simulink library "pwrsysBasic"  (R2016a)
settings: Solver=VariableStepAuto  SolverMode=SingleTasking  StartTime=0.0  StopTime=10.0  RelTol=1e-3
values from neighbouring files (symbols this model uses):
  Ts = Ts_c    (= 1e-07)    [PlantStateEquations_abc_Script.m]
undefined symbols (not defined in the file or in its folder): DiscIntNeverNeededParam, fn, Iap, Uanp
undefined symbols (not defined in the file): Sn, tctrl
libraries: pwrsysBasic x15, powerlib_meascontrol x12, pwrsysTransf x8, simulink x2
(part 1 of 2)
settings Model: Creator=daniemot  LastModifiedBy=daniemot
settings DebuggingCC: SFUnexpectedBacktrackingDiag=error  SFNoUnconditionalDefaultTransitionDiag=error
settings GRTTargetCC: TargetLangStandard=C99 (ISO)  GeneratePreprocessorConditionals=Use local settings
settings ConfigComp: CovMetricSettings=dwe  CovHtmlReporting=off  CovSaveCumulativeToWorkspaceVar=off  CovSaveSingleToWorkspaceVar=off  CovExternalEMLEnable=on

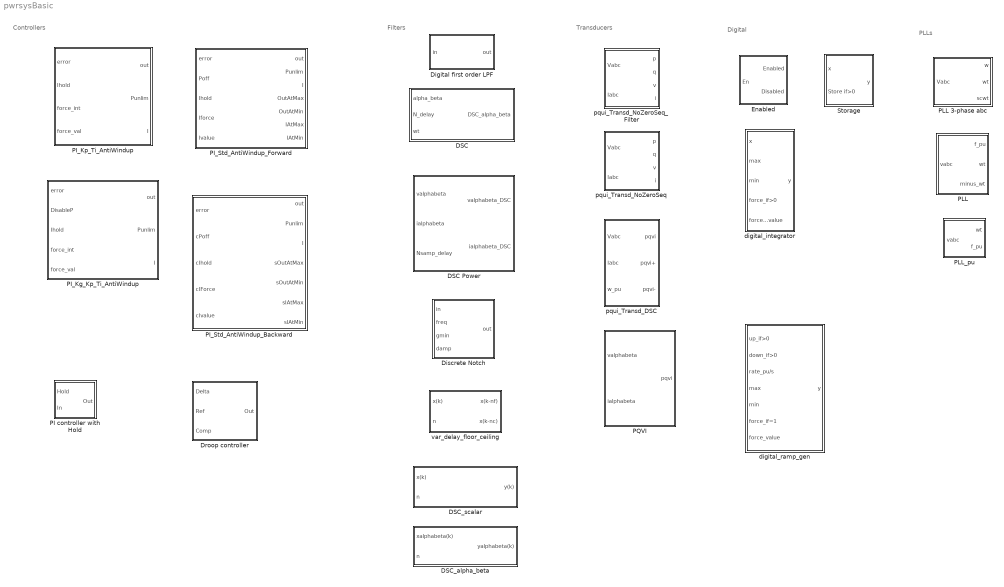
== system pwrsysBasic ==
  note: PLLs
  note: Controllers
  note: Filters
  note: Transducers
  note: Digital
  DSC : Subsystem
  "DSC Power " : Subsystem
  DSC_alpha_beta : Subsystem  mask(Delayed signal cancellation of a scalar){nmax=200}
      mask prompts: nmax "Circular buffer size"
      mask help: Performs an adaptive delayed signal cancellation of the input x. The input n should be equal to (floating point) number of samples corresponding to half the period of the frequency f one intends to filter.
      mask Help:
      | Performs two delayed signal cancellation of the input x:
      | 	yf(k) = 0.5 (x(k) + x(k-nf(k))
      | 	yc(k) = 0.5 (x(k) + x(k-nc(k))
      | where, f stands for floor and c for ceiling.
      | 
      | The two values yf and yc are then weigthed according to how far the real value n is from nc or nf.
      | 
      | Inputs:
      | 	x: input signal
      | 	n: floating point representing the number of samples equal to half the period of the frequecy one intends to suppress
      | 
      | Output:
      | 	y: output with the delayed signal cancelled value of the input
      | 
      | Parameter:
      | 	Circular buffer size: set to the number of samples that corresponds to half the period of the lowest frequency one intends to filter.
      | 
      | States:
      | 	Uses an S-function with a circular buffer that supplies the delayed (ceiling and floor of n) values of the input.
      mask Display: fprintf('DSC');
  DSC_scalar : Subsystem  mask(Delayed signal cancellation of a scalar){nmax=200}
      mask prompts: nmax "Circular buffer size"
      mask help: Performs an adaptive delayed signal cancellation of the input x. The input n should be equal to (floating point) number of samples corresponding to half the period of the frequency f one intends to filter.
      mask Help:
      | Performs two delayed signal cancellation of the input x:
      | 	yf(k) = 0.5 (x(k) + x(k-nf(k))
      | 	yc(k) = 0.5 (x(k) + x(k-nc(k))
      | where, f stands for floor and c for ceiling.
      | 
      | The two values yf and yc are then weigthed according to how far the real value n is from nc or nf.
      | 
      | Inputs:
      | 	x: input signal
      | 	n: floating point representing the number of samples equal to half the period of the frequecy one intends to suppress
      | 
      | Output:
      | 	y: output with the delayed signal cancelled value of the input
      | 
      | Parameter:
      | 	Circular buffer size: set to the number of samples that corresponds to half the period of the lowest frequency one intends to filter.
      | 
      | States:
      | 	Uses an S-function with a circular buffer that supplies the delayed (ceiling and floor of n) values of the input.
      mask Display: fprintf('y(k)=0.5(x(k) + x(k-n))');
  Digital first order LPF : Subsystem  mask(Digital first-order low-pass filter){Ts=tctrl, fcutout=fn/2^0.5}
      mask prompts: Ts "Sample times [s]"; fcutout "Cutout frequency [Hz]"
      mask help:
      | Continuous time transfer function:  1/(1 + s T)
      | 	where T [s] = 1 / (2 pi fcutout [Hz]).
      |
      | Actual digital transfer function:   alpha / (1 + ( alpha -1) z^{-1} )
      | 	with eq. of diffs.: y = alpha x + (1 - alpha) y z^{-1}
      | 	where alpha = Ts / ( 1/(2 pi fcutout) + Ts)
      mask Display: fprintf('1/(1+sT)');
  Discrete Notch : Subsystem  TreatAsAtomicUnit=on  mask(Discrete Notch with time-varying parameters){Ts=0.001}
      mask prompts: Ts "Sample time Ts (s)"
      mask help:
      | The block implements the Tustin discretization of a continuous-time notch filter with time-varying coefficients:
      | (s^2+2*gmin*damp*freq*s+freq^2)/(s^2+2*damp*freq*s+freq^2)
      |
      | Parameters:
      | - freq is the notch frequency (rad/s)
      | - gmin is the minimum gain
      | - damp is the damping ratio
      mask Display: fprintf('notch');
  Droop controller : Subsystem  mask(Droop controller){Refmax=1, Refmin=-1, Ts=-1, Kp=1, Kd=0, Tr=0.1, flp=100, DB=0}
      mask prompts: Refmax "Max reference"; Refmin "Min reference"; Ts "Sample time"; Kp "Permanent gain"; Kd "Transient gain"; Tr "Reset time [s]"; flp "Low-pass filter cut-off frequency [Hz]"; DB "Dead-band"
      mask help:
      | This block implements a droop controller, i.e. it provides compensation of the input Ref based on the input Delta and Comp.
      |
      | The input Delta is used as input of a PD controller which provides permanent (proportional) and transient (derivative) droop of the input Ref.
      |
      | The input Comp divides the output value of the droop controller and may be used for other types of compensation.
      mask DialogControl DescTextVar Prompt: This block implements a simplified model for power control with droop influence. It can be used either for active power with frequency droop influence or reactive power with voltage droop influence.
  Enabled : Subsystem  SystemSampleTime=Ts  mask(Enabled block){}
      mask help:
      | if En > 0
      |     Enabled = 1;
      |     Disabled = 0;
      | else
      |     Enabled = 0;
      |     Disabled = 1;
      | end
      mask Display: fprintf('Enable');
  PI controller with Hold : Subsystem  mask(PI controller with anti-windup){Kp=1, Ki=0, Max=1, Min=-1, x0=0, Ts=1e-4}
      mask prompts: Kp "Proportional gain"; Ki "Integral gain"; Max "Maximum output"; Min "Minimum output"; x0 "Initial condition"; Ts "Sampling time"
      mask help:
      | This block implements a PI controller with anti-windup
      |
      | The input hold freezes the integrator and allows implementing anti-windup in control loops with feed-forward or dynamic limits
  PI_Kg_Kp_Ti_AntiWindup : Subsystem  TreatAsAtomicUnit=on  SystemSampleTime=Ts  mask(PI regulator with anti-windup){Ts=0.001, Kg=1, Kp=1, Ti=1, PI_max=1, PI_min=-1}
      mask prompts: Ts "Sampling time [s]"; Kg "Loop gain: Kg [pu]"; Kp "Proportional gain: Kp [pu]"; Ti "Integral time: Ti [s]"; PI_max "Maximum output [pu]"; PI_min "Minimum output [pu]"
      mask help:
      | Discrete PI regulator with forward Euler approximation for the integrator.
      |
      | Transfer function:
      | 	Kg (Kp + 1/sTi)
      |
      | The anti-windup freezes the integrator if the unlimited output of the PI goes beyond the limits.
      |
      | It is possible to disable the proportional (Kp) contribution.
      settings: MinAlgLoopOccurrences=on
      mask Display: fprintf('Kg(Kp+1/(sTi))');
  PI_Kp_Ti_AntiWindup : Subsystem  TreatAsAtomicUnit=on  SystemSampleTime=Ts  mask(PI regulator with anti-windup){Ts=0.001, Kp=10, Ti=1, PI_max=1, PI_min=-1}
      mask prompts: Ts "Sampling time [s]"; Kp "Proportional gain: Kp [pu]"; Ti "Integral time: Ti [s]"; PI_max "Maximum output [pu]"; PI_min "Minimum output [pu]"
      mask help:
      | Discrete PI regulator with forward Euler approximation for the integrator.
      |
      | Transfer function:
      | 	Kp (1 + sTi) / (sTi)
      |
      | The anti-windup freezes the integrator if the unlimited output of the PI goes beyond the limits.
      settings: MinAlgLoopOccurrences=on
      mask Display: fprintf('Kp(1+1/(sTi))');
  PI_Std_AntiWindup_Backward : Subsystem  mask(PI regulator with anti-windup){Ts=1, Kg=1, Kp=1, Ti=1, outMax=1, outMin=1}
      mask prompts: Ts "Sampling time [s]"; Kg "Loop gain Kg [pu]"; Kp "Proportional gain Kp [pu]"; Ti "Integral time Ti [s]"; outMax "Maximum output [pu]"; outMin "Minimum output [pu]"
      mask help:
      | Discrete PI regulator in standard form with loop gain and backward Euler approximation.
      |
      | Transfer function:
      | 	Kg (Kp + 1/sTi)
      |
      | The anti-windup freezes the integrator if the unlimited output of the PI goes beyond the limits.
      |
      | It is possible to:
      | - Disable the proportional (Kp) contribution. (Poff > 0)
      | - Freeze the integrator (Ihold >0)
      | - Force the integrator to Ivalue (Iforce >0)
      mask Display: fprintf('Kg(Kp+1/(sTi))');
  PI_Std_AntiWindup_Forward : Subsystem  SystemSampleTime=Ts  mask(PI regulator with anti-windup){Ts=0.001, Kg=1, Kp=1, Ti=1, outMax=1, outMin=-1}
      mask prompts: Ts "Sampling time [s]"; Kg "Loop gain: Kg [pu]"; Kp "Proportional gain: Kp [pu]"; Ti "Integral time: Ti [s]"; outMax "Maximum output [pu]"; outMin "Minimum output [pu]"
      mask help:
      | Discrete PI regulator in standard form with loop gain and forward Euler method  for the integrator.
      |
      | Transfer function:
      | 	Kg (Kp + 1/sTi)
      |
      | The anti-windup freezes the integrator if the unlimited output of the PI goes beyond the limits.
      |
      | It is possible to:
      | - Disable the proportional (Kp) contribution. (Poff > 0)
      | - Freeze the integrator (Ihold >0)
      | - Force the integrator to Ivalue (Iforce >0)
      settings: MinAlgLoopOccurrences=on
      mask Display: fprintf('Kg(Kp+1/(sTi))');
  PLL : Subsystem  mask(Matlabs PLL with POS and NEG omega t output){fn=0, Ts=0.00005, Kp_pll=90, Ki_pll=1600, Kd_pll=0, PLL_ini=0}
      mask prompts: fn "Rated frequency [Hz]"; Ts "Sampling time [s]"; Kp_pll "Proportional gain: Kp_pll"; Ki_pll "Integral gain: Ki_pll"; Kd_pll "Derivative gain: Kd_pll"; PLL_ini "PLL initial angle: PLL_ini [degrees]"
  PLL 3-phase abc : Subsystem  mask(3-Phase PLL in the abc frame){fnom=50, fdev=20, zeta=0.707, Kp=100, Ki=50, Kd=1e4, Tr=100, Ts=1e-4, wt0=0}
      mask prompts: fnom "Rated frequency [Hz]"; fdev "Maximum frequency deviation [Hz]"; zeta "Damping ratio"; Kp "Proportional gain"; Ki "Integral gain"; Kd "Derivative gain"; Tr "Reset time [s]"; Ts "Sampling time [s]"; wt0 "Initial angle [rad/s]"
      mask help: This block implements a 3-phase PLL in the abc reference frame.
      mask init:
      | wn = fnom/(4*zeta);
      mask DialogControl freqFilter Prompt: Frequency filter
      mask DialogControl ctrl Prompt: Controller
  PLL_pu : Subsystem  mask(Matlabs PLL with POS and NEG omega t output){fn=50, Ts=100e-6, Kp_pll=90, Ki_pll=1600, Kd_pll=0, PLL_ini=0}
      mask prompts: fn "Rated frequency [Hz]"; Ts "Sampling time [s]"; Kp_pll "Proportional gain: Kp_pll"; Ki_pll "Integral gain: Ki_pll"; Kd_pll "Derivative gain: Kd_pll"; PLL_ini "PLL initial angle: PLL_ini [degrees]"
  PQVI : Subsystem  mask(u i p q transducer - No zero sequence){Sn=Sn, Uanp=Uanp, Iap=Iap}
      mask prompts: Sn "Rated three-phase apparent power [VA]"; Uanp "Rated peak phase-to-groud voltage [V]"; Iap "Rated peak line current [A]"
      mask help:
      | Loosely based on Akagi 1984, but with Clarke Transformation for both the current and voltage
      | 	v  = (valpha^2 + vbeta^2)^0.5 / V_phase_peak
      | 	i   = (ialpha^2 + ibeta^2)^0.5 / I_line_peak
      | 	p  = 3/2 * (valpha ialpha +vbeta ibeta) / Sn
      | 	q  = 3/2 * (-valpha ibeta +vbeta ialpha) / Sn
  Storage : Subsystem  SystemSampleTime=Ts  mask(Storage block){}
      mask help:
      | if Store ==1
      |     Output = Input;
      | else
      |     Output = old ouptut;
      | end
      mask Display: fprintf('Store');
  digital_integrator : Subsystem  SystemSampleTime=Ts  mask(Digital integrator){Ts=Ts}
      mask prompts: Ts "Sample times [s]"
      mask help:
      | Forward Euler method: as in matlab help
      | 	y(n) = y(n-1) + Ts(n-1)*x(n-1)
      | uset it to avoid algebraic loops
      |
      | All inputs are stored in states, so there is no direct feedthrough. GAMBIARRA for avoiding algebraic loops, see https://www.mathworks.com/help/simulink/ug/integration-considerations-for-matlab-function-blocks.html
      |
      | Inputs
      |    x: input to the integrator
      |    max: max value for integrator
      |    min: min value for integrator
      |    force: if>=1 sets integrator to forceval
      |    forceval: see line above (max and min are respected
      |    Ts: sampling time
      | Output
      |    y: output of the integrator
      mask Display: fprintf('1/s');
  digital_ramp_gen : Subsystem  SystemSampleTime=Ts  mask(Digital ramp generator){Ts=tctrl}
      mask prompts: Ts "Sample times [s]"
      mask help: Allways starts at zero. Can be forced to a value, and will stay there, but in the first two cycles will stay at zero.
      mask Display: fprintf('Ramp');
  pqui_Transd_DSC : Subsystem  mask(DSC u i p q transducer - No zero sequence){Ts=0.000005, fn=50, Sn=Sn, Uanp=Uanp, Iap=Iap}
      mask prompts: Ts "Sampling time [s]"; fn "Rated frequency [Hz]"; Sn "Rated three-phase apparent power [VA]"; Uanp "Rated peak phase-to-groud voltage [V]"; Iap "Rated peak line current [A]"
      mask help:
      | Loosely based on Akagi 1984, but with Clarke Transformation for both the current and voltage
      | 	v  = (valpha^2 + vbeta^2)^0.5 / V_phase_peak
      | 	i   = (ialpha^2 + ibeta^2)^0.5 / I_line_peak
      | 	p  = 3/2 * (valpha ialpha +vbeta ibeta) / Sn
      | 	q  = 3/2 * (-valpha ibeta +vbeta ialpha) / Sn
  pqui_Transd_NoZeroSeq : Subsystem  mask(u i p q transducer - No zero sequence){Sn=Sn, Uanp=Uanp, Iap=Iap}
      mask prompts: Sn "Rated three-phase apparent power [VA]"; Uanp "Rated peak phase-to-groud voltage [V]"; Iap "Rated peak line current [A]"
      mask help:
      | Loosely based on Akagi 1984, but with Clarke Transformation for both the current and voltage
      | 	v  = (valpha^2 + vbeta^2)^0.5 / V_phase_peak
      | 	i   = (ialpha^2 + ibeta^2)^0.5 / I_line_peak
      | 	p  = 3/2 * (valpha ialpha +vbeta ibeta) / Sn
      | 	q  = 3/2 * (-valpha ibeta +vbeta ialpha) / Sn
  pqui_Transd_NoZeroSeq_Filter : Subsystem  mask(u i p q transducer - No zero sequence){Ts=0.001, Sn=1000, fn=50, Uanp=1000, Iap=1000, fcutoutvi=1000, fcutoutpq=1000, zeta=0.7}
      mask prompts: Ts "Sampling time [s]"; Sn "Rated three-phase apparent power [VA]"; fn "Rated frequency [Hz]"; Uanp "Rated peak phase-to-groud voltage [V]"; Iap "Rated peak line current [A]"; fcutoutvi "Cutout freq. low-pass for v&i meas. [Hz]"; fcutoutpq "Cutout freq. low-pass for p&q meas. [Hz]"; zeta "Zeta for all second order filters"
      mask help:
      | Loosely based on Akagi 1984, but with Clarke Transformation for both the current and voltage
      | 	v  = (valpha^2 + vbeta^2)^0.5 / V_phase_peak
      | 	i   = (ialpha^2 + ibeta^2)^0.5 / I_line_peak
      | 	p  = 3/2 * (valpha ialpha +vbeta ibeta) / Sn
      | 	q  = 3/2 * (-valpha ibeta +vbeta ialpha) / Sn
      |
      | Second order low-pass filter for all measurements
      |
      | Notch filter at the rated frequency
  var_delay_floor_ceiling : Subsystem  mask(Circular buffer with two variable delays (ceiling and floor)){nmax=40}
      mask prompts: nmax "Circular buffer size"
      mask help: Provides the values of the input delayed by floor(n) and ceil(n) samples.
      mask Help:
      | Provides the values of the input delayed by floor(n) and ceil(n) samples.
      | 
      | S-Function source code:
      | 	variable_delay_floor_ceil.c
      | 	variable_delay_floor_ceil_wrapper.c
      | 	variable_delay_floor_ceil.tlc
      | 
      | mexw64:
      | 	variable_delay_floor_ceil.mexw64
      | 
      | The mex file can be regenerated by running this at the command line:
      | 	mex variable_delay_floor_ceil.c variable_delay_floor_ceil_wrapper.c
      | This assumes that the addons for compiling are installed.

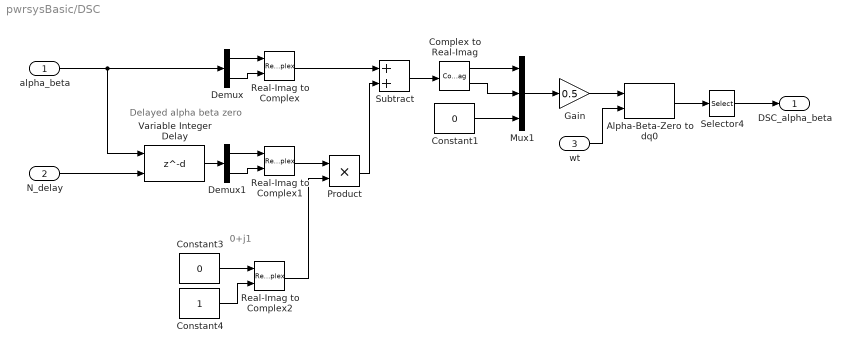
== system pwrsysBasic/DSC ==
  note: 0+j1
  note: Delayed alpha beta zero
  alpha_beta : Inport
  N_delay : Inport  Port=2
  wt : Inport  Port=3
  Alpha-Beta-Zero to dq0 : powerlib_meascontrol/Transformations/Alpha-Beta-Zero to dq0  Alignment=90 degrees behind phase A axis
  Complex to Real-Imag : ComplexToRealImag
  Constant1 : Constant  Value=0
  Constant3 : Constant  Value=0
  Constant4 : Constant
  Demux : Demux  Outputs=2
  Demux1 : Demux  Outputs=2
  Gain : Gain  Gain=0.5
  Mux1 : Mux  Inputs=[1 1 1]
  Product : Product
  Real-Imag to Complex : RealImagToComplex
  Real-Imag to Complex1 : RealImagToComplex
  Real-Imag to Complex2 : RealImagToComplex
  Selector4 : Selector  InputPortWidth=3  IndexOptions=Index vector (dialog)  Indices=[1 2]  OutputSizes=1
  Subtract : Sum
  Variable Integer Delay : Delay  DelayLengthSource=Input port  DelayLength=200  DelayLengthUpperLimit=500  SampleTime=Ts
      settings: InputPortMap=u0,p1
  DSC_alpha_beta : Outport
  wires:
  Product/1 -> Subtract/2
  Demux/1 -> Real-Imag to Complex/1
  Real-Imag to Complex1/1 -> Product/1
  Demux1/1 -> Real-Imag to Complex1/1
  wt/1 -> Alpha-Beta-Zero to dq0/2
  Complex to Real-Imag/1 -> Mux1/1
  Variable Integer Delay/1 -> Demux1/1
  Demux1/2 -> Real-Imag to Complex1/2
  N_delay/1 -> Variable Integer Delay/2
  Gain/1 -> Alpha-Beta-Zero to dq0/1
  Constant3/1 -> Real-Imag to Complex2/1
  Real-Imag to Complex/1 -> Subtract/1
  alpha_beta/1 -> Variable Integer Delay/1, Demux/1
  Real-Imag to Complex2/1 -> Product/2
  Subtract/1 -> Complex to Real-Imag/1
  Constant1/1 -> Mux1/3
  Demux/2 -> Real-Imag to Complex/2
  Constant4/1 -> Real-Imag to Complex2/2
  Complex to Real-Imag/2 -> Mux1/2
  Mux1/1 -> Gain/1
  Alpha-Beta-Zero to dq0/1 -> Selector4/1
  Selector4/1 -> DSC_alpha_beta/1

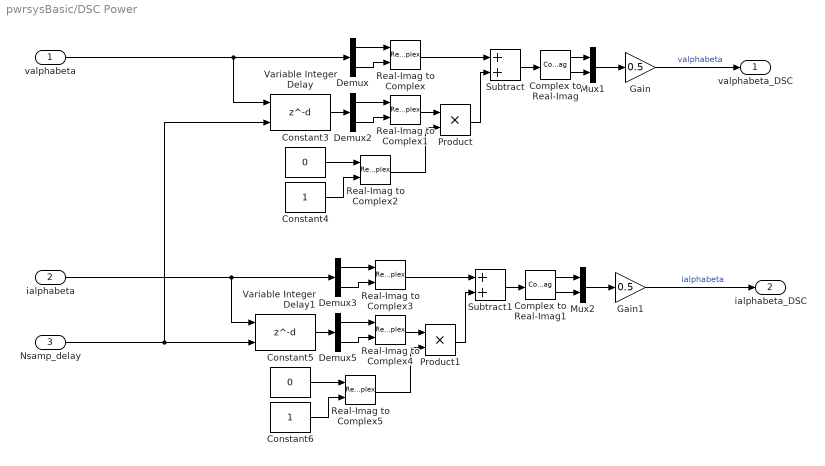
== system pwrsysBasic/DSC Power  ==
  valphabeta : Inport
  ialphabeta : Inport  Port=2
  Nsamp_delay : Inport  Port=3
  Complex to Real-Imag : ComplexToRealImag
  Complex to Real-Imag1 : ComplexToRealImag
  Constant3 : Constant  Value=0
  Constant4 : Constant
  Constant5 : Constant  Value=0
  Constant6 : Constant
  Demux{,2..3,5} (4 alike) : Demux  Outputs=2
  Gain : Gain  Gain=0.5
  Gain1 : Gain  Gain=0.5
  Mux1 : Mux  Inputs=[1 1]
  Mux2 : Mux  Inputs=[1 1]
  Product : Product
  Product1 : Product
  Real-Imag to Complex{,1..5} (6 alike) : RealImagToComplex
  Subtract : Sum
  Subtract1 : Sum
  Variable Integer Delay : Delay  DelayLengthSource=Input port  DelayLength=200  DelayLengthUpperLimit=500  SampleTime=Ts
      settings: InputPortMap=u0,p1
  Variable Integer Delay1 : Delay  DelayLengthSource=Input port  DelayLength=200  DelayLengthUpperLimit=500  SampleTime=Ts
      settings: InputPortMap=u0,p1
  valphabeta_DSC : Outport
  ialphabeta_DSC : Outport  Port=2
  wires:
  Demux2/2 -> Real-Imag to Complex1/2
  Demux3/1 -> Real-Imag to Complex3/1
  Constant6/1 -> Real-Imag to Complex5/2
  Constant5/1 -> Real-Imag to Complex5/1
  Real-Imag to Complex5/1 -> Product1/2
  Complex to Real-Imag1/1 -> Mux2/1
  Real-Imag to Complex4/1 -> Product1/1
  Demux3/2 -> Real-Imag to Complex3/2
  Gain1/1 -> ialphabeta_DSC/1  "ialphabeta"
  Complex to Real-Imag1/2 -> Mux2/2
  Complex to Real-Imag/1 -> Mux1/1
  Mux2/1 -> Gain1/1
  valphabeta/1 -> Demux/1, Variable Integer Delay/1
  Real-Imag to Complex2/1 -> Product/2
  Subtract1/1 -> Complex to Real-Imag1/1
  Real-Imag to Complex3/1 -> Subtract1/1
  Mux1/1 -> Gain/1
  Constant3/1 -> Real-Imag to Complex2/1
  Demux/1 -> Real-Imag to Complex/1
  Variable Integer Delay1/1 -> Demux5/1
  Demux5/2 -> Real-Imag to Complex4/2
  Demux2/1 -> Real-Imag to Complex1/1
  Variable Integer Delay/1 -> Demux2/1
  Product/1 -> Subtract/2
  Nsamp_delay/1 -> Variable Integer Delay1/2, Variable Integer Delay/2
  Complex to Real-Imag/2 -> Mux1/2
  Product1/1 -> Subtract1/2
  Gain/1 -> valphabeta_DSC/1  "valphabeta"
  Real-Imag to Complex1/1 -> Product/1
  Real-Imag to Complex/1 -> Subtract/1
  Subtract/1 -> Complex to Real-Imag/1
  Constant4/1 -> Real-Imag to Complex2/2
  ialphabeta/1 -> Demux3/1, Variable Integer Delay1/1
  Demux5/1 -> Real-Imag to Complex4/1
  Demux/2 -> Real-Imag to Complex/2

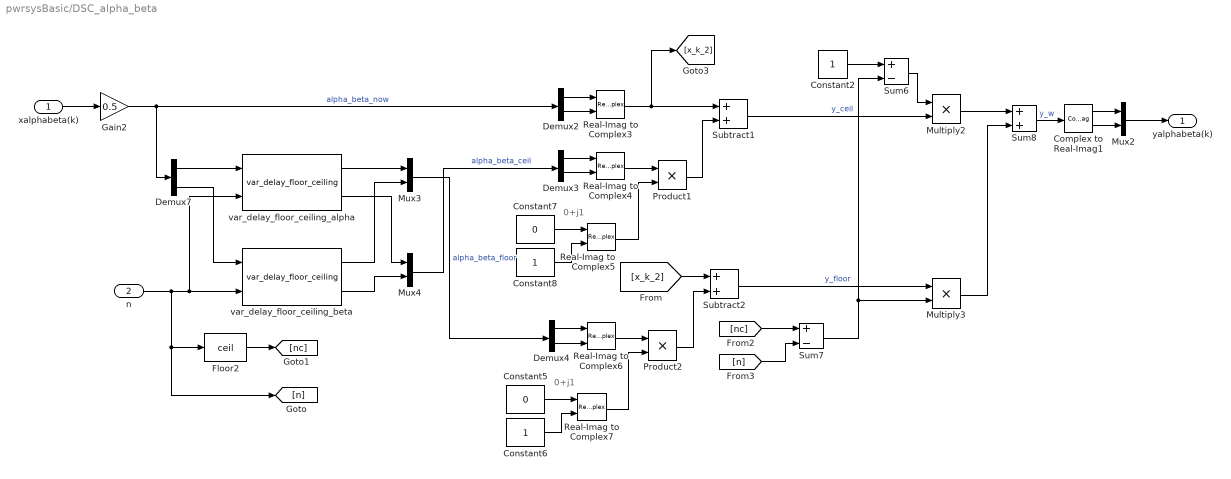
== system pwrsysBasic/DSC_alpha_beta ==
  note: 0+j1
  note: 0+j1
  xalphabeta(k) : Inport
  n : Inport  Port=2
  Complex to Real-Imag1 : ComplexToRealImag
  Constant2 : Constant
  Constant5 : Constant  Value=0
  Constant6 : Constant
  Constant7 : Constant  Value=0
  Constant8 : Constant
  Demux{2..4,7} (4 alike) : Demux  Outputs=2
  Floor2 : Rounding  Operator=ceil
  Gain2 : Gain  Gain=0.5
  Multiply2 : Product
  Multiply3 : Product
  Mux2 : Mux  Inputs=[1 1]
  Mux3 : Mux  Inputs=[1 1]
  Mux4 : Mux  Inputs=[1 1]
  Product1 : Product
  Product2 : Product
  Real-Imag to Complex{3..7} (5 alike) : RealImagToComplex
  Subtract1 : Sum
  Subtract2 : Sum
  Sum6 : Sum  Inputs=+-
  Sum7 : Sum  Inputs=+-
  Sum8 : Sum
  var_delay_floor_ceiling_alpha : pwrsysBasic/var_delay_floor_ceiling  nmax=nmax
  var_delay_floor_ceiling_beta : pwrsysBasic/var_delay_floor_ceiling  nmax=nmax
  yalphabeta(k) : Outport
  wires:
  Complex to Real-Imag1/2 -> Mux2/2
  Mux2/1 -> yalphabeta(k)/1
  Demux2/1 -> Real-Imag to Complex3/1
  Product1/1 -> Subtract1/2
  xalphabeta(k)/1 -> Gain2/1
  Demux2/2 -> Real-Imag to Complex3/2
  Mux4/1 -> Demux3/1  "alpha_beta_ceil"
  Complex to Real-Imag1/1 -> Mux2/1
  Demux3/2 -> Real-Imag to Complex4/2
  Constant8/1 -> Real-Imag to Complex5/2
  n/1 -> var_delay_floor_ceiling_alpha/2, var_delay_floor_ceiling_beta/2, Floor2/1, [n]
  Real-Imag to Complex3/1 -> [x_k_2], Subtract1/1
  Constant7/1 -> Real-Imag to Complex5/1
  Real-Imag to Complex4/1 -> Product1/1
  Demux3/1 -> Real-Imag to Complex4/1
  Real-Imag to Complex5/1 -> Product1/2
  [nc] -> Sum7/1
  Sum7/1 -> Multiply3/2, Sum6/2
  Subtract2/1 -> Multiply3/1  "y_floor"
  Subtract1/1 -> Multiply2/2  "y_ceil"
  Multiply2/1 -> Sum8/1
  Multiply3/1 -> Sum8/2
  Sum6/1 -> Multiply2/1
  [n] -> Sum7/2
  Constant2/1 -> Sum6/1
  Floor2/1 -> [nc]
  Demux4/1 -> Real-Imag to Complex6/1
  Constant5/1 -> Real-Imag to Complex7/1
  Demux4/2 -> Real-Imag to Complex6/2
  Constant6/1 -> Real-Imag to Complex7/2
  Product2/1 -> Subtract2/2
  Real-Imag to Complex6/1 -> Product2/1
  Real-Imag to Complex7/1 -> Product2/2
  Mux3/1 -> Demux4/1  "alpha_beta_floor"
  Gain2/1 -> Demux7/1, Demux2/1  "alpha_beta_now"
  [x_k_2] -> Subtract2/1
  Sum8/1 -> Complex to Real-Imag1/1  "y_w"
  Demux7/1 -> var_delay_floor_ceiling_alpha/1
  Demux7/2 -> var_delay_floor_ceiling_beta/1
  var_delay_floor_ceiling_alpha/1 -> Mux3/1
  var_delay_floor_ceiling_beta/1 -> Mux3/2
  var_delay_floor_ceiling_alpha/2 -> Mux4/1
  var_delay_floor_ceiling_beta/2 -> Mux4/2

== system pwrsysBasic/DSC_scalar ==
  x(k) : Inport
  n : Inport  Port=2
  Constant : Constant
  Floor1 : Rounding  Operator=ceil
  Gain : Gain  Gain=0.5
  Multiply : Product
  Multiply1 : Product
  Sum1 : Sum  Inputs=+-
  Sum2 : Sum  Inputs=+-
  Sum3 : Sum
  Sum4 : Sum
  Sum5 : Sum
  var_delay_floor_ceiling : pwrsysBasic/var_delay_floor_ceiling  nmax=nmax
  y(k) : Outport
  wires:
  x(k)/1 -> Gain/1
  Sum3/1 -> Multiply/2  "y_ceil"
  Sum4/1 -> Multiply1/1  "y_floor"
  Constant/1 -> Sum1/1
  Sum2/1 -> Multiply1/2, Sum1/2
  Floor1/1 -> Sum2/1
  n/1 -> var_delay_floor_ceiling/2, Sum2/2, Floor1/1
  Multiply1/1 -> Sum5/2
  Multiply/1 -> Sum5/1
  Sum1/1 -> Multiply/1
  Gain/1 -> var_delay_floor_ceiling/1, Sum4/1, Sum3/1
  Sum5/1 -> y(k)/1  "y_w"
  var_delay_floor_ceiling/1 -> Sum3/2
  var_delay_floor_ceiling/2 -> Sum4/2

== system pwrsysBasic/Digital first order LPF ==
  note: Transfer function: alpha / ( 1 + ( alpha -1 ) z^{-1} )
  note: alpha = Ts / ( 1/(2 pi fcutout) + Ts )
  note: y = alpha x + ( 1 - alpha) y z^{-1}
  in : Inport
  Discrete Filter : DiscreteFilter  Numerator=[Ts/(1/(2*pi*fcutout)+Ts)]  Denominator=[1 Ts/(1/(2*pi*fcutout)+Ts)-1]  SampleTime=Ts
  Rate Transition3 : RateTransition  OutPortSampleTime=Ts
  out : Outport
  wires:
  in/1 -> Rate Transition3/1
  Rate Transition3/1 -> Discrete Filter/1
  Discrete Filter/1 -> out/1

== system pwrsysBasic/Discrete Notch ==
  in : Inport
  freq : Inport  Port=2
  gmin : Inport  Port=3
  damp : Inport  Port=4
  S-Function Builder : S-Function  InitFcn=try, set_param(gcb,'FunctionName','notch'), end  FunctionName=notch  Parameters=Ts  SFunctionModules=notch_wrapper  SFunctionDeploymentMode=off  EnableBusSupport=off  mask(S-Function Builder){}
      mask help: Simulink:masks:SFunctionBuilder_MD
      mask init:
      | val = [[.9  0.75 0.75 1 1 .9 .9 1]',[1 1 0.75 0.75 .9 .9 1 .9]'];try , sys = get_param(gcb,'SfunBuilderFcnName');if isempty(sys), sys = get_param(gcb,'FunctionName'); end,catch, sys = get_param(gcb,'FunctionName'); end
      settings: PreSaveFcn=try, set_param(gcb,'FunctionName','notch'), end  OpenFcn=sfunctionwizard(gcbh)
      mask Display: plot(val(:,1),val(:,2)),disp(sys), port_label('input',1,'in'), port_label('input',2,'freq'), port_label('input',3,'gmin'), port_label('input',4,'damp'), port_label('output',1,'out')
  out : Outport
  wires:
  in/1 -> S-Function Builder/1
  freq/1 -> S-Function Builder/2
  gmin/1 -> S-Function Builder/3
  damp/1 -> S-Function Builder/4
  S-Function Builder/1 -> out/1

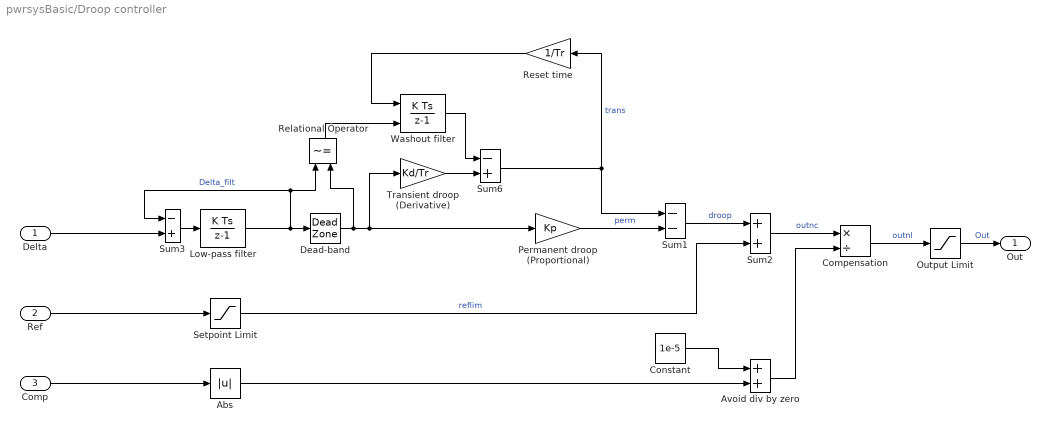
== system pwrsysBasic/Droop controller ==
  Delta : Inport
  Ref : Inport  Port=2
  Comp : Inport  Port=3
  Abs : Abs  ZeroCross=off
  Avoid div by zero : Sum
  Compensation : Product  Inputs=*/
  Constant : Constant  Value=1e-5  SampleTime=Ts
  Dead-band : DeadZone  LowerValue=-DB  UpperValue=DB  SaturateOnIntegerOverflow=on
  Low-pass filter : DiscreteIntegrator  gainval=flp  InitialConditionSetting=State (most efficient)  SampleTime=Ts  UpperSaturationLimit=Refmax/Kp  LowerSaturationLimit=Refmin/Kp  ICPrevOutput=DiscIntNeverNeededParam  ICPrevScaledInput=DiscIntNeverNeededParam
  Output Limit : Saturate  UpperLimit=Refmax  LowerLimit=Refmin  ZeroCross=off
  Permanent droop (Proportional) : Gain  Gain=Kp
  Relational Operator : RelationalOperator  Operator=~=  OutDataTypeStr=boolean
  Reset time : Gain  Gain=1/Tr
  Setpoint Limit : Saturate  UpperLimit=Refmax  LowerLimit=Refmin  ZeroCross=off
  Sum1 : Sum  Inputs=--
  Sum2 : Sum
  Sum3 : Sum  Inputs=-+
  Sum6 : Sum  Inputs=-+
  Transient droop (Derivative) : Gain  Gain=Kd/Tr
  Washout filter : DiscreteIntegrator  gainval=1  ExternalReset=level  InitialConditionSetting=State (most efficient)  SampleTime=Ts  LimitOutput=on  UpperSaturationLimit=Refmax  LowerSaturationLimit=Refmin  ICPrevOutput=DiscIntNeverNeededParam  ICPrevScaledInput=DiscIntNeverNeededParam
  Out : Outport
  wires:
  Permanent droop (Proportional)/1 -> Sum1/2  "perm"
  Washout filter/1 -> Sum6/1
  Transient droop (Derivative)/1 -> Sum6/2
  Sum1/1 -> Sum2/1  "droop"
  Sum6/1 -> Sum1/1, Reset time/1  "trans"
  Reset time/1 -> Washout filter/1
  Sum2/1 -> Compensation/1  "outnc"
  Dead-band/1 -> Relational Operator/2, Permanent droop (Proportional)/1, Transient droop (Derivative)/1
  Setpoint Limit/1 -> Sum2/2  "reflim"
  Constant/1 -> Avoid div by zero/1
  Avoid div by zero/1 -> Compensation/2
  Output Limit/1 -> Out/1  "Out"
  Abs/1 -> Avoid div by zero/2
  Relational Operator/1 -> Washout filter/2
  Compensation/1 -> Output Limit/1  "outnl"
  Sum3/1 -> Low-pass filter/1
  Low-pass filter/1 -> Relational Operator/1, Sum3/1, Dead-band/1  "Delta_filt"
  Delta/1 -> Sum3/2
  Ref/1 -> Setpoint Limit/1
  Comp/1 -> Abs/1

== system pwrsysBasic/Enabled ==
  En : Inport
  S-Function Builder : S-Function  InitFcn=try, set_param(gcb,'FunctionName','enabled'), end  FunctionName=enabled  SFunctionModules=enabled_wrapper  SFunctionDeploymentMode=off  EnableBusSupport=off  mask(S-Function Builder){}
      mask help: Simulink:masks:SFunctionBuilder_MD
      mask init: same as pwrsysBasic/Discrete Notch/S-Function Builder
      settings: PreSaveFcn=try, set_param(gcb,'FunctionName','enabled'), end  OpenFcn=sfunctionwizard(gcbh)
      mask Display: plot(val(:,1),val(:,2)),disp(sys), port_label('input',1,'En'), port_label('output',1,'Enabled'), port_label('output',2,'Disabled')
  Enabled : Outport
  Disabled : Outport  Port=2
  wires:
  En/1 -> S-Function Builder/1
  S-Function Builder/1 -> Enabled/1
  S-Function Builder/2 -> Disabled/1

== system pwrsysBasic/PI controller with Hold ==
  Hold : Inport
  In : Inport  Port=2
  Anti-windup : Switch  Criteria=u2 ~= 0
  Discrete-Time Integrator : DiscreteIntegrator  InitialCondition=x0  InitialConditionSetting=State (most efficient)  SampleTime=Ts  UpperSaturationLimit=Max  LowerSaturationLimit=Min  ICPrevOutput=DiscIntNeverNeededParam  ICPrevScaledInput=DiscIntNeverNeededParam
  Eq. 10-X4 : Sum  SaturateOnIntegerOverflow=on  InputSameDT=on  OutDataTypeStr=Inherit: Same as first input
  Integral : Gain  Gain=Ki
  Logical Operator : Logic  Operator=OR  AllPortsSameDT=off  OutDataTypeStr=boolean
  Proportional : Gain  Gain=Kp
  Relational Operator : RelationalOperator  Operator=~=  OutDataTypeStr=boolean
  Saturation : Saturate  UpperLimit=Max  LowerLimit=Min
  v1 : Constant  Value=0
  Out : Outport
  wires:
  Discrete-Time Integrator/1 -> Eq. 10-X4/2
  Integral/1 -> Anti-windup/3
  Anti-windup/1 -> Discrete-Time Integrator/1
  Hold/1 -> Logical Operator/1
  In/1 -> Integral/1, Proportional/1
  Eq. 10-X4/1 -> Saturation/1, Relational Operator/1
  v1/1 -> Anti-windup/1
  Saturation/1 -> Relational Operator/2, Out/1
  Logical Operator/1 -> Anti-windup/2
  Proportional/1 -> Eq. 10-X4/1
  Relational Operator/1 -> Logical Operator/2

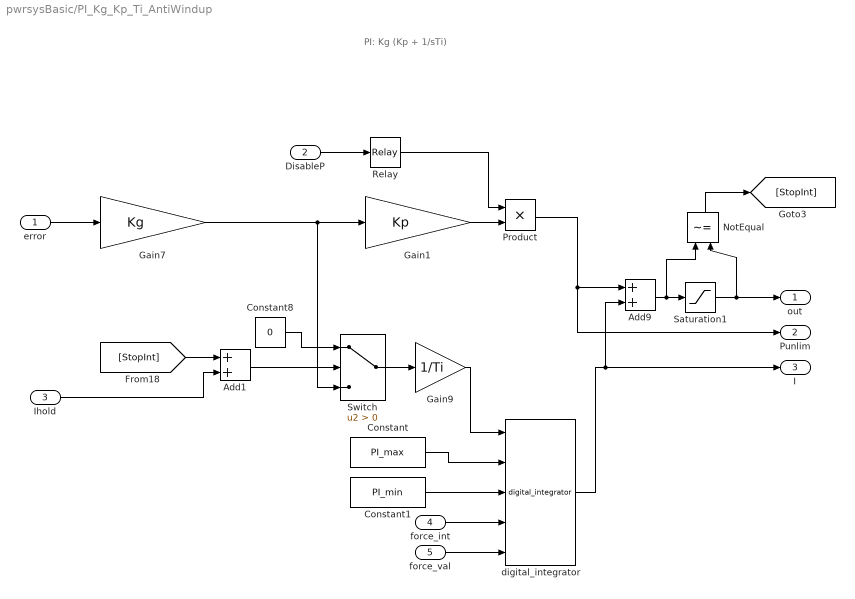
== system pwrsysBasic/PI_Kg_Kp_Ti_AntiWindup ==
  note: PI: Kg (Kp + 1/sTi)
  error : Inport
  DisableP : Inport  Port=2
  Ihold : Inport  Port=3
  force_int : Inport  Port=4
  force_val : Inport  Port=5
  Add1 : Sum
  Add9 : Sum
  Constant : Constant  Value=PI_max
  Constant1 : Constant  Value=PI_min
  Constant8 : Constant  Value=0
  Gain1 : Gain  Gain=Kp
  Gain7 : Gain  Gain=Kg
  Gain9 : Gain  Gain=1/Ti
  NotEqual : RelationalOperator  Operator=~=  OutDataTypeStr=boolean
  Product : Product
  Relay : Relay  OnSwitchValue=0.6  OffSwitchValue=0.4  OnOutputValue=0  OffOutputValue=1
  Saturation1 : Saturate  UpperLimit=PI_max  LowerLimit=PI_min
  Switch : Switch  Criteria=u2 > Threshold
  digital_integrator : pwrsysBasic/digital_integrator  Ts=Ts
  out : Outport
  Punlim : Outport  Port=2
  I : Outport  Port=3
  wires:
  NotEqual/1 -> [StopInt]
  Saturation1/1 -> out/1, NotEqual/2
  error/1 -> Gain7/1
  digital_integrator/1 -> I/1, Add9/2
  Add1/1 -> Switch/2
  Constant8/1 -> Switch/1
  Gain7/1 -> Gain1/1, Switch/3
  Switch/1 -> Gain9/1
  Add9/1 -> NotEqual/1, Saturation1/1
  Gain9/1 -> digital_integrator/1
  [StopInt] -> Add1/1
  Ihold/1 -> Add1/2
  Product/1 -> Punlim/1, Add9/1
  Gain1/1 -> Product/2
  DisableP/1 -> Relay/1
  Relay/1 -> Product/1
  force_val/1 -> digital_integrator/5
  force_int/1 -> digital_integrator/4
  Constant1/1 -> digital_integrator/3
  Constant/1 -> digital_integrator/2

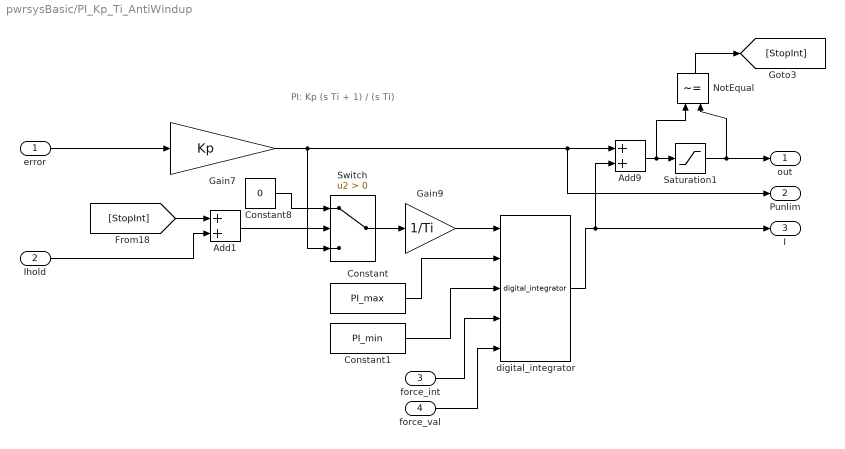
== system pwrsysBasic/PI_Kp_Ti_AntiWindup ==
  note: PI: Kp (s Ti + 1) / (s Ti)
  error : Inport
  Ihold : Inport  Port=2
  force_int : Inport  Port=3
  force_val : Inport  Port=4
  Add1 : Sum
  Add9 : Sum
  Constant : Constant  Value=PI_max
  Constant1 : Constant  Value=PI_min
  Constant8 : Constant  Value=0
  Gain7 : Gain  Gain=Kp
  Gain9 : Gain  Gain=1/Ti
  NotEqual : RelationalOperator  Operator=~=  OutDataTypeStr=boolean
  Saturation1 : Saturate  UpperLimit=PI_max  LowerLimit=PI_min
  Switch : Switch  Criteria=u2 > Threshold
  digital_integrator : pwrsysBasic/digital_integrator  Ts=Ts
  out : Outport
  Punlim : Outport  Port=2
  I : Outport  Port=3
  wires:
  NotEqual/1 -> [StopInt]
  Saturation1/1 -> out/1, NotEqual/2
  error/1 -> Gain7/1
  digital_integrator/1 -> I/1, Add9/2
  Add1/1 -> Switch/2
  Constant8/1 -> Switch/1
  Gain7/1 -> Switch/3, Punlim/1, Add9/1
  Switch/1 -> Gain9/1
  Add9/1 -> NotEqual/1, Saturation1/1
  Gain9/1 -> digital_integrator/1
  [StopInt] -> Add1/1
  Ihold/1 -> Add1/2
  Constant1/1 -> digital_integrator/3
  force_int/1 -> digital_integrator/4
  force_val/1 -> digital_integrator/5
  Constant/1 -> digital_integrator/2

== system pwrsysBasic/PI_Std_AntiWindup_Backward ==
  error : Inport
  cPoff : Inport  Port=2
  cIhold : Inport  Port=3
  cIForce : Inport  Port=4
  cIvalue : Inport  Port=5
  Data Type Conversion1 : DataTypeConversion  OutDataTypeStr=double
  Data Type Conversion2 : DataTypeConversion  OutDataTypeStr=double
  Data Type Conversion4 : DataTypeConversion  OutDataTypeStr=double
  S-Function Builder : S-Function  InitFcn=try, set_param(gcb,'FunctionName','pi_std_antiwindup'), end  FunctionName=pi_std_antiwindup  Parameters=Ts,Kg,Kp,Ti,outMax,outMin  SFunctionModules=pi_std_antiwindup_wrapper  SFunctionDeploymentMode=off  EnableBusSupport=off  mask(S-Function Builder){}
      mask help: Simulink:masks:SFunctionBuilder_MD
      mask init: same as pwrsysBasic/Discrete Notch/S-Function Builder
      settings: PreSaveFcn=try, set_param(gcb,'FunctionName','pi_std_antiwindup'), end  OpenFcn=sfunctionwizard(gcbh)
      mask Display: plot(val(:,1),val(:,2)),disp(sys), port_label('input',1,'error'), port_label('input',2,'cPoff'), port_label('input',3,'cIhold'), port_label('input',4,'cIforce'), port_label('input',5,'Ivalue'), port_label('output',1,'out'), port_label('output',2,'sOutAtMax'), port_label('output',3,'sOutAtMin'), port_label('output',4,'sIAtMax'), port_label('output',5,'sIAtMin'), port_label('output',6,'Punlim'), port_label('output',7,'I')
  out : Outport
  Punlim : Outport  Port=2
  I : Outport  Port=3
  sOutAtMax : Outport  Port=4
  sOutAtMin : Outport  Port=5
  sIAtMax : Outport  Port=6
  sIAtMin : Outport  Port=7
  wires:
  Data Type Conversion1/1 -> S-Function Builder/2
  Data Type Conversion2/1 -> S-Function Builder/3
  Data Type Conversion4/1 -> S-Function Builder/4
  error/1 -> S-Function Builder/1
  cPoff/1 -> Data Type Conversion1/1
  cIhold/1 -> Data Type Conversion2/1
  cIForce/1 -> Data Type Conversion4/1
  cIvalue/1 -> S-Function Builder/5
  S-Function Builder/5 -> sIAtMin/1
  S-Function Builder/6 -> Punlim/1
  S-Function Builder/7 -> I/1
  S-Function Builder/3 -> sOutAtMin/1
  S-Function Builder/1 -> out/1
  S-Function Builder/2 -> sOutAtMax/1
  S-Function Builder/4 -> sIAtMax/1

== system pwrsysBasic/PI_Std_AntiWindup_Forward ==
  note: PI: Kg (Kp + 1/sTi)
  error : Inport
  Poff : Inport  Port=2
  Ihold : Inport  Port=3
  Iforce : Inport  Port=4
  Ivalue : Inport  Port=5
  Data Type Conversion1 : DataTypeConversion  OutDataTypeStr=double
  Data Type Conversion2 : DataTypeConversion  OutDataTypeStr=double
  Data Type Conversion4 : DataTypeConversion  OutDataTypeStr=double
  S-Function Builder : S-Function  InitFcn=try, set_param(gcb,'FunctionName','pi_std_antiwindup'), end  FunctionName=pi_std_antiwindup  Parameters=Ts,Kg,Kp,Ti,outMax,outMin  SFunctionModules=pi_std_antiwindup_wrapper  SFunctionDeploymentMode=off  EnableBusSupport=off  mask(S-Function Builder){}
      mask help: Simulink:masks:SFunctionBuilder_MD
      mask init: same as pwrsysBasic/Discrete Notch/S-Function Builder
      settings: PreSaveFcn=try, set_param(gcb,'FunctionName','pi_std_antiwindup'), end  OpenFcn=sfunctionwizard(gcbh)
      mask Display: plot(val(:,1),val(:,2)),disp(sys), port_label('input',1,'error'), port_label('input',2,'cPoff'), port_label('input',3,'cIhold'), port_label('input',4,'cIforce'), port_label('input',5,'Ivalue'), port_label('output',1,'out'), port_label('output',2,'sOutAtMax'), port_label('output',3,'sOutAtMin'), port_label('output',4,'sIAtMax'), port_label('output',5,'sIAtMin'), port_label('output',6,'Punlim'), port_label('output',7,'I')
  out : Outport
  Punlim : Outport  Port=2
  I : Outport  Port=3
  OutAtMax : Outport  Port=4
  OutAtMin : Outport  Port=5
  IAtMax : Outport  Port=6
  IAtMin : Outport  Port=7
  wires:
  Data Type Conversion1/1 -> S-Function Builder/2
  Data Type Conversion2/1 -> S-Function Builder/3
  Data Type Conversion4/1 -> S-Function Builder/4
  error/1 -> S-Function Builder/1
  Poff/1 -> Data Type Conversion1/1
  Ihold/1 -> Data Type Conversion2/1
  Iforce/1 -> Data Type Conversion4/1
  Ivalue/1 -> S-Function Builder/5
  S-Function Builder/1 -> out/1
  S-Function Builder/2 -> OutAtMax/1
  S-Function Builder/3 -> OutAtMin/1
  S-Function Builder/4 -> IAtMax/1
  S-Function Builder/5 -> IAtMin/1
  S-Function Builder/6 -> Punlim/1
  S-Function Builder/7 -> I/1

== system pwrsysBasic/PLL ==
  vabc : Inport
  PLL (3ph) : powerlib_meascontrol/PLL/PLL (3ph)  Fmin=0.8*fn  Par_Init=[PLL_ini, fn]  ParK=[Kp_pll, Ki_pll, Kd_pll]  TcD=1e-4  MaxRateChangeFreq=fn/5  FilterCutOffFreq=fn/2  Ts=Ts  AGC=on
  Rate Transition1 : RateTransition  OutPortSampleTime=Ts
  Rtot_pu1 : Gain  Gain=-1  SaturateOnIntegerOverflow=on  OutDataTypeStr=Inherit: Same as input  ParamDataTypeStr=Inherit: Same as input
  Rtot_pu3 : Gain  Gain=1/fn  SaturateOnIntegerOverflow=on  OutDataTypeStr=Inherit: Same as input  ParamDataTypeStr=Inherit: Same as input
  f_pu : Outport
  wt : Outport  Port=2
  minus_wt : Outport  Port=3
  wires:
  Rtot_pu3/1 -> f_pu/1
  vabc/1 -> Rate Transition1/1
  Rate Transition1/1 -> PLL (3ph)/1
  PLL (3ph)/2 -> Rtot_pu1/1, wt/1
  PLL (3ph)/1 -> Rtot_pu3/1
  Rtot_pu1/1 -> minus_wt/1

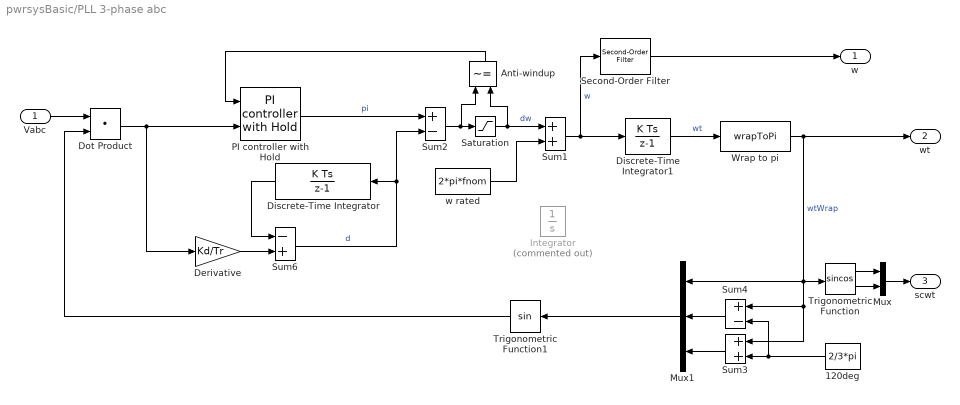
== system pwrsysBasic/PLL 3-phase abc ==
  Vabc : Inport
  120deg : Constant  Value=2/3*pi  SampleTime=Ts
  Anti-windup : RelationalOperator  Operator=~=  OutDataTypeStr=boolean
  Derivative : Gain  Gain=Kd/Tr
  Discrete-Time Integrator : DiscreteIntegrator  gainval=1/Tr  InitialConditionSetting=State (most efficient)  SampleTime=Ts  LimitOutput=on  UpperSaturationLimit=2*pi*fdev  LowerSaturationLimit=-2*pi*fdev  ICPrevOutput=DiscIntNeverNeededParam  ICPrevScaledInput=DiscIntNeverNeededParam
  Discrete-Time Integrator1 : DiscreteIntegrator  gainval=1  InitialCondition=wt0  InitialConditionSetting=State (most efficient)  SampleTime=Ts  UpperSaturationLimit=2*pi*fdev  LowerSaturationLimit=-2*pi*fdev  ICPrevOutput=DiscIntNeverNeededParam  ICPrevScaledInput=DiscIntNeverNeededParam
  Dot Product : DotProduct  InputSameDT=on  OutDataTypeStr=Inherit: Inherit via internal rule
  Integrator : Integrator  Commented=on  InitialCondition=wt0  UpperSaturationLimit=1  LowerSaturationLimit=-1  ZeroCross=off
  Mux : Mux  Inputs=2
  Mux1 : Mux  Inputs=3
  PI controller with Hold : pwrsysBasic/PI controller  with Hold  Kp=Kp  Ki=Ki  Max=2*pi*fdev  Min=-2*pi*fdev  x0=0  Ts=Ts
  Saturation : Saturate  UpperLimit=2*pi*fdev  LowerLimit=-2*pi*fdev
  Second-Order Filter : powerlib_meascontrol/Filters/Second-Order Filter  FilterType=Lowpass  Fo=wn  Zeta=zeta  Ts=Ts  Initialize=on  Vac_Init="[0,  0,  60]"  Vdc_Init=2*pi*fnom  PlotResponse=off  FreqRange=[0, 500, 1]
  Sum1 : Sum
  Sum2 : Sum  Inputs=+-
  Sum3 : Sum
  Sum4 : Sum  Inputs=+-
  Sum6 : Sum  Inputs=-+
  Trigonometric Function : Trigonometry  Operator=sincos  ApproximationMethod=CORDIC
  Trigonometric Function1 : Trigonometry  ApproximationMethod=CORDIC
  Wrap to pi : MATLABFcn  MATLABFcn=wrapToPi
  w rated : Constant  Value=2*pi*fnom  SampleTime=Ts
  w : Outport
  wt : Outport  Port=2
  scwt : Outport  Port=3
  wires:
  Discrete-Time Integrator/1 -> Sum6/1
  Sum6/1 -> Discrete-Time Integrator/1, Sum2/2  "d"
  Derivative/1 -> Sum6/2
  Saturation/1 -> Sum1/1, Anti-windup/2  "dw"
  w rated/1 -> Sum1/2
  Sum1/1 -> Discrete-Time Integrator1/1, Second-Order Filter/1  "w"
  Discrete-Time Integrator1/1 -> Wrap to pi/1  "wt"
  Vabc/1 -> Dot Product/1
  PI controller with Hold/1 -> Sum2/1  "pi"
  Sum2/1 -> Anti-windup/1, Saturation/1
  Wrap to pi/1 -> Mux1/1, Trigonometric Function/1, Sum4/1, Sum3/1, wt/1  "wtWrap"
  Trigonometric Function/1 -> Mux/1
  Trigonometric Function/2 -> Mux/2
  Mux/1 -> scwt/1
  120deg/1 -> Sum4/2, Sum3/2
  Sum4/1 -> Mux1/2
  Sum3/1 -> Mux1/3
  Mux1/1 -> Trigonometric Function1/1
  Trigonometric Function1/1 -> Dot Product/2
  Second-Order Filter/1 -> w/1
  Dot Product/1 -> Derivative/1, PI controller with Hold/2
  Anti-windup/1 -> PI controller with Hold/1

== system pwrsysBasic/PLL_pu ==
  vabc : Inport
  PLL (3ph) : powerlib_meascontrol/PLL/PLL (3ph)  Fmin=0.8*fn  Par_Init=[PLL_ini, fn]  ParK=[Kp_pll, Ki_pll, Kd_pll]  TcD=1e-3  MaxRateChangeFreq=fn/5  FilterCutOffFreq=fn/2  Ts=Ts  AGC=on
  Rate Transition1 : RateTransition  OutPortSampleTime=Ts
  Rtot_pu3 : Gain  Gain=1/fn  SaturateOnIntegerOverflow=on  OutDataTypeStr=Inherit: Same as input  ParamDataTypeStr=Inherit: Same as input
  wt : Outport
  f_pu : Outport  Port=2
  wires:
  Rtot_pu3/1 -> f_pu/1
  vabc/1 -> Rate Transition1/1
  Rate Transition1/1 -> PLL (3ph)/1
  PLL (3ph)/2 -> wt/1
  PLL (3ph)/1 -> Rtot_pu3/1

== system pwrsysBasic/PQVI ==
  note: Akagi 1984 for p and q
      | calc. without zero seq,
      | factor 3/2 compensates for
      | amplitude invariant
      | Clarke transformation
  valphabeta : Inport
  ialphabeta : Inport  Port=2
  Add3 : Sum  Inputs=+-
  Bus Creator : BusCreator  Inputs=4
  Demux1 : Demux  Outputs=2
  Demux4 : Demux  Outputs=2
  Dot Product : DotProduct  InputSameDT=on  OutDataTypeStr=Inherit: Inherit via internal rule
  Gain1 : Gain  Gain=3/2/Sn
  Gain2 : Gain  Gain=3/2/Sn
  Gain3 : Gain  Gain=1/Uanp
  Gain4 : Gain  Gain=1/Iap
  Hypot : Math  Operator=hypot  RndMeth=Zero  SaturateOnIntegerOverflow=on
  Hypot1 : Math  Operator=hypot  RndMeth=Zero  SaturateOnIntegerOverflow=on
  Product3 : Product
  Product4 : Product
  pqvi : Outport
  wires:
  Gain4/1 -> Bus Creator/4  "i"
  Gain1/1 -> Bus Creator/1  "p"
  Gain2/1 -> Bus Creator/2  "q"
  Product4/1 -> Add3/2
  Dot Product/1 -> Gain1/1  "p"
  Hypot1/1 -> Gain4/1  "i"
  Gain3/1 -> Bus Creator/3  "v"
  Demux1/2 -> Hypot1/2, Product4/2
  valphabeta/1 -> Demux4/1, Dot Product/1
  Demux1/1 -> Hypot1/1, Product3/2
  ialphabeta/1 -> Demux1/1, Dot Product/2
  Add3/1 -> Gain2/1  "q"
  Demux4/2 -> Hypot/2, Product3/1
  Product3/1 -> Add3/1
  Hypot/1 -> Gain3/1  "v"
  Demux4/1 -> Hypot/1, Product4/1
  Bus Creator/1 -> pqvi/1

== system pwrsysBasic/Storage ==
  x : Inport
  Store if>0 : Inport  Port=2
  S-Function Builder : S-Function  InitFcn=try, set_param(gcb,'FunctionName','store'), end  FunctionName=store  SFunctionModules=store_wrapper  SFunctionDeploymentMode=off  EnableBusSupport=off  mask(S-Function Builder){}
      mask help: Simulink:masks:SFunctionBuilder_MD
      mask init: same as pwrsysBasic/Discrete Notch/S-Function Builder
      settings: PreSaveFcn=try, set_param(gcb,'FunctionName','store'), end  OpenFcn=sfunctionwizard(gcbh)
      mask Display: plot(val(:,1),val(:,2)),disp(sys), port_label('input',1,'u'), port_label('input',2,'store'), port_label('output',1,'y')
  y : Outport
  wires:
  S-Function Builder/1 -> y/1
  x/1 -> S-Function Builder/1
  Store if>0/1 -> S-Function Builder/2

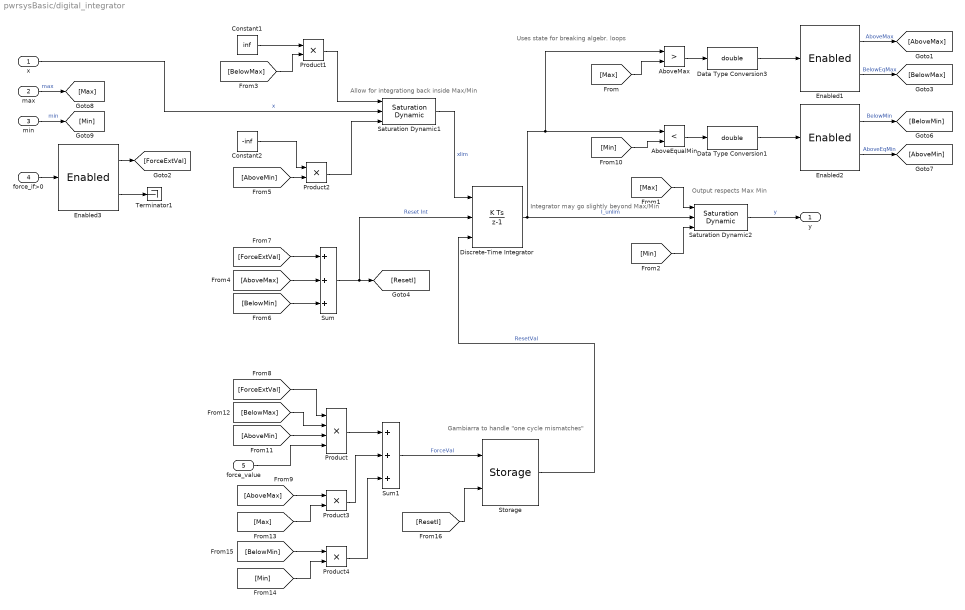
== system pwrsysBasic/digital_integrator ==
  note: Gambiarra to handle "one cycle mismatches"
  note: Integrator may go slightly beyond Max/Min
  note: Output respects Max Min
  note: Uses state for breaking algebr. loops
  note: Allow for integrationg back inside Max/Min
  x : Inport
  max : Inport  Port=2
  min : Inport  Port=3
  force_if>0 : Inport  Port=4
  force_value : Inport  Port=5
  AboveEqualMin : RelationalOperator  Operator=<  OutDataTypeStr=boolean
  AboveMax : RelationalOperator  Operator=>  OutDataTypeStr=boolean
  Constant1 : Constant  Value=inf
  Constant2 : Constant  Value=-inf
  Data Type Conversion1 : DataTypeConversion  OutDataTypeStr=double
  Data Type Conversion3 : DataTypeConversion  OutDataTypeStr=double
  Discrete-Time Integrator : DiscreteIntegrator  ExternalReset=level  InitialConditionSource=external  InitialConditionSetting=State (most efficient)  SampleTime=Ts  IgnoreLimit=on  ICPrevOutput=DiscIntNeverNeededParam  ICPrevScaledInput=DiscIntNeverNeededParam
  Enabled1 : pwrsysBasic/Basic Blocks/Enabled
  Enabled2 : pwrsysBasic/Enabled
  Enabled3 : pwrsysBasic/Enabled
  Product : Product  Inputs=4
  Product{1..4} (4 alike) : Product
  Saturation Dynamic1 : simulink/Discontinuities/Saturation Dynamic  OutMin=[]  OutMax=[]  OutDataTypeStr=Inherit: Same as second input  OutDataType=fixdt(1, 16)  OutScaling=2^-10  DoSatur=off
  Saturation Dynamic2 : simulink/Discontinuities/Saturation Dynamic  OutMin=[]  OutMax=[]  OutDataTypeStr=Inherit: Same as second input  OutDataType=fixdt(1, 16)  OutScaling=2^-10  DoSatur=off
  Storage : pwrsysBasic/Storage
  Sum : Sum  Inputs=+++
  Sum1 : Sum  Inputs=+++
  Terminator1 : Terminator
  y : Outport
  wires:
  x/1 -> Saturation Dynamic1/2  "x"
  Saturation Dynamic2/1 -> y/1  "y"
  max/1 -> [Max]  "max"
  min/1 -> [Min]  "min"
  force_value/1 -> Product/4
  Saturation Dynamic1/1 -> Discrete-Time Integrator/1  "xlim"
  [BelowMax] -> Product1/2
  Constant1/1 -> Product1/1
  Product1/1 -> Saturation Dynamic1/1
  [AboveMin] -> Product2/2
  Constant2/1 -> Product2/1
  Product2/1 -> Saturation Dynamic1/3
  Enabled1/1 -> [AboveMax]  "AboveMax"
  Enabled1/2 -> [BelowMax]  "BelowEqMax"
  Enabled2/2 -> [AboveMin]  "AboveEqMin"
  Enabled2/1 -> [BelowMin]  "BelowMin"
  [AboveMax] -> Sum/2
  [BelowMin] -> Sum/3
  force_if>0/1 -> Enabled3/1
  Enabled3/2 -> Terminator1/1
  [ForceExtVal] -> Product/1
  [AboveMax] -> Product3/1
  [Min] -> AboveEqualMin/2
  [AboveMin] -> Product/3
  [BelowMax] -> Product/2
  Product/1 -> Sum1/1
  [Max] -> Product3/2
  [BelowMin] -> Product4/1
  [Min] -> Product4/2
  Product4/1 -> Sum1/3
  Product3/1 -> Sum1/2
  Sum1/1 -> Storage/1  "ForceVal"
  Enabled3/1 -> [ForceExtVal]
  [Max] -> AboveMax/2
  Discrete-Time Integrator/1 -> Saturation Dynamic2/2, AboveEqualMin/1, AboveMax/1  "I_unlim"
  [Max] -> Saturation Dynamic2/1
  [Min] -> Saturation Dynamic2/3
  AboveMax/1 -> Data Type Conversion3/1
  AboveEqualMin/1 -> Data Type Conversion1/1
  Data Type Conversion3/1 -> Enabled1/1
  Data Type Conversion1/1 -> Enabled2/1
  [ForceExtVal] -> Sum/1
  Sum/1 -> Discrete-Time Integrator/2, [ResetI]  "Reset Int"
  [ResetI] -> Storage/2
  Storage/1 -> Discrete-Time Integrator/3  "ResetVal"

== system pwrsysBasic/digital_ramp_gen ==
  up_if>0 : Inport
  down_if>0 : Inport  Port=2
  rate_pu/s : Inport  Port=3
  max : Inport  Port=4
  min : Inport  Port=5
  force_if=1 : Inport  Port=6
  force_value : Inport  Port=7
  Constant : Constant  Value=Ts
  MATLAB Function : MATLAB Function  TreatAsAtomicUnit=on  SystemSampleTime=Ts
      settings: RTWSystemCode=Inline
  y : Outport
  wires:
  up_if>0/1 -> MATLAB Function/1(up)
  MATLAB Function/1(y) -> y/1
  max/1 -> MATLAB Function/4(max)
  min/1 -> MATLAB Function/5(min)
  force_if=1/1 -> MATLAB Function/6(force)
  force_value/1 -> MATLAB Function/7(forceval)
  Constant/1 -> MATLAB Function/8(Ts)
  down_if>0/1 -> MATLAB Function/2(down)
  rate_pu/s/1 -> MATLAB Function/3(rate)

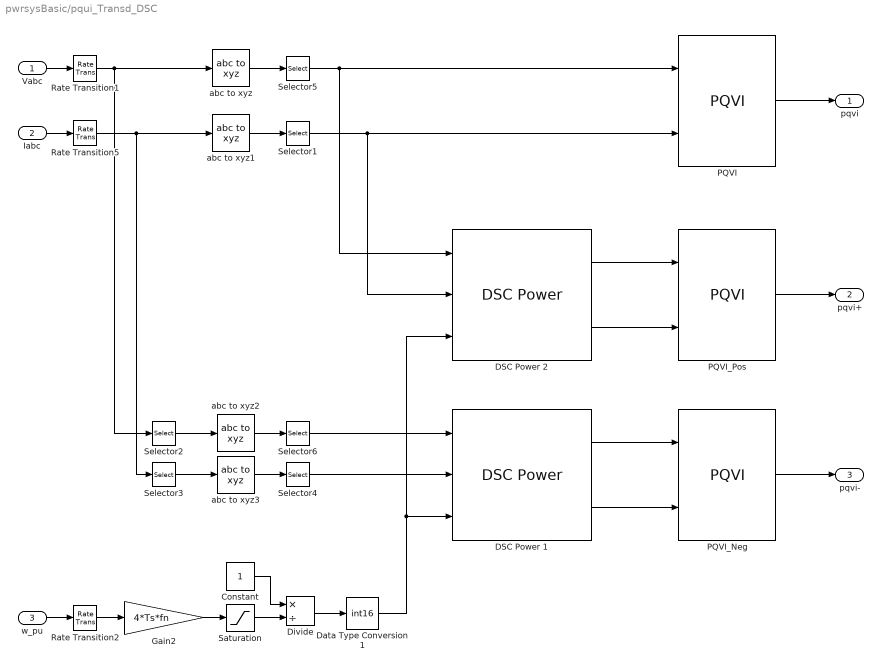
== system pwrsysBasic/pqui_Transd_DSC ==
  Vabc : Inport
  Iabc : Inport  Port=2
  w_pu : Inport  Port=3
  Constant : Constant
  DSC Power 1 : pwrsysBasic/DSC Power 
  DSC Power 2 : pwrsysBasic/DSC Power 
  Data Type Conversion1 : DataTypeConversion  OutDataTypeStr=int16  RndMeth=Round  SaturateOnIntegerOverflow=on
  Divide : Product  Inputs=*/
  Gain2 : Gain  Gain=4*Ts*fn
  PQVI : pwrsysBasic/PQVI  Sn=Sn  Uanp=Uanp  Iap=Iap
  PQVI_Neg : pwrsysBasic/PQVI  Sn=Sn  Uanp=Uanp  Iap=Iap
  PQVI_Pos : pwrsysBasic/PQVI  Sn=Sn  Uanp=Uanp  Iap=Iap
  Rate Transition1 : RateTransition  OutPortSampleTime=Ts
  Rate Transition2 : RateTransition  X0=1  OutPortSampleTime=Ts
  Rate Transition5 : RateTransition  OutPortSampleTime=Ts
  Saturation : Saturate  UpperLimit=inf  LowerLimit=0.000001
  Selector{1,4..6} (4 alike) : Selector  InputPortWidth=3  IndexOptions=Index vector (dialog)  Indices=[1 2]  OutputSizes=1
  Selector2 : Selector  InputPortWidth=3  IndexOptions=Index vector (dialog)  Indices=[1 3 2]  OutputSizes=1
  Selector3 : Selector  InputPortWidth=3  IndexOptions=Index vector (dialog)  Indices=[1 3 2]  OutputSizes=1
  abc to xyz{,1..3} (4 alike) : pwrsysTransf/abc to xyz  typeTransf=Amplitude-invariant
  pqvi : Outport
  pqvi+ : Outport  Port=2
  pqvi- : Outport  Port=3
  wires:
  abc to xyz1/1 -> Selector1/1
  Vabc/1 -> Rate Transition1/1
  Iabc/1 -> Rate Transition5/1
  Rate Transition1/1 -> abc to xyz/1, Selector2/1
  Rate Transition5/1 -> abc to xyz1/1, Selector3/1
  Selector5/1 -> DSC Power 2/1, PQVI/1
  Selector1/1 -> DSC Power 2/2, PQVI/2
  PQVI/1 -> pqvi/1
  Data Type Conversion1/1 -> DSC Power 1/3, DSC Power 2/3
  DSC Power 2/1 -> PQVI_Pos/1
  DSC Power 2/2 -> PQVI_Pos/2
  PQVI_Pos/1 -> pqvi+/1
  abc to xyz2/1 -> Selector6/1
  abc to xyz3/1 -> Selector4/1
  Selector2/1 -> abc to xyz2/1
  Selector3/1 -> abc to xyz3/1
  Selector6/1 -> DSC Power 1/1
  Selector4/1 -> DSC Power 1/2
  PQVI_Neg/1 -> pqvi-/1
  DSC Power 1/2 -> PQVI_Neg/2
  DSC Power 1/1 -> PQVI_Neg/1
  Saturation/1 -> Divide/2
  Constant/1 -> Divide/1
  Rate Transition2/1 -> Gain2/1
  w_pu/1 -> Rate Transition2/1
  Gain2/1 -> Saturation/1
  Divide/1 -> Data Type Conversion1/1
  abc to xyz/1 -> Selector5/1

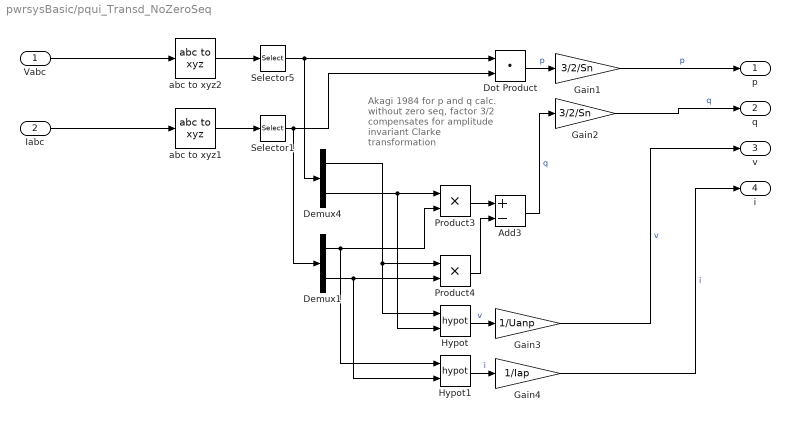
== system pwrsysBasic/pqui_Transd_NoZeroSeq ==
  note: Akagi 1984 for p and q
      | calc. without zero seq,
      | factor 3/2 compensates for
      | amplitude invariant
      | Clarke transformation
  Vabc : Inport
  Iabc : Inport  Port=2
  Add3 : Sum  Inputs=+-
  Demux1 : Demux  Outputs=2
  Demux4 : Demux  Outputs=2
  Dot Product : DotProduct  InputSameDT=on  OutDataTypeStr=Inherit: Inherit via internal rule
  Gain1 : Gain  Gain=3/2/Sn
  Gain2 : Gain  Gain=3/2/Sn
  Gain3 : Gain  Gain=1/Uanp
  Gain4 : Gain  Gain=1/Iap
  Hypot : Math  Operator=hypot  RndMeth=Zero  SaturateOnIntegerOverflow=on
  Hypot1 : Math  Operator=hypot  RndMeth=Zero  SaturateOnIntegerOverflow=on
  Product3 : Product
  Product4 : Product
  Selector1 : Selector  InputPortWidth=3  IndexOptions=Index vector (dialog)  Indices=[1 2]  OutputSizes=1
  Selector5 : Selector  InputPortWidth=3  IndexOptions=Index vector (dialog)  Indices=[1 2]  OutputSizes=1
  abc to xyz1 : pwrsysTransf/abc to xyz  typeTransf=Amplitude-invariant
  abc to xyz2 : pwrsysTransf/abc to xyz  typeTransf=Amplitude-invariant
  p : Outport
  q : Outport  Port=2
  v : Outport  Port=3
  i : Outport  Port=4
  wires:
  abc to xyz1/1 -> Selector1/1
  Gain3/1 -> v/1  "v"
  Demux1/2 -> Hypot1/2, Product4/2
  Hypot1/1 -> Gain4/1  "i"
  Selector1/1 -> Demux1/1, Dot Product/2
  Selector5/1 -> Demux4/1, Dot Product/1
  Demux4/1 -> Hypot/1, Product4/1
  Hypot/1 -> Gain3/1  "v"
  Dot Product/1 -> Gain1/1  "p"
  Demux1/1 -> Hypot1/1, Product3/2
  Add3/1 -> Gain2/1  "q"
  Product4/1 -> Add3/2
  Demux4/2 -> Hypot/2, Product3/1
  Vabc/1 -> abc to xyz2/1
  abc to xyz2/1 -> Selector5/1
  Iabc/1 -> abc to xyz1/1
  Product3/1 -> Add3/1
  Gain1/1 -> p/1  "p"
  Gain4/1 -> i/1  "i"
  Gain2/1 -> q/1  "q"
